simulink model "DC_observer_R2018a"  (R2018a)
settings: Solver=VariableStepAuto  StartTime=0.0  StopTime=2  MaxStep=1e-4  RelTol=1e-3
values from neighbouring files (symbols this model uses):
  A = [ -(k*gr)^2/(J*R)-b/J, 0 ... (first row only)    [DC_statespace.m]    (also in DC_statespace_facit.m; DC_statespace_observer.m)
  b = 20    [DC_statespace.m]    (also in DC_statespace_facit.m; DC_statespace_observer.m = B(1,1))
  B = [k*gr/(J*R) ... (first row only)    [DC_statespace.m]    (also in DC_statespace_facit.m; DC_statespace_observer.m)
  C = [0, 1]    [DC_statespace.m]    (also in DC_statespace_facit.m; DC_statespace_observer.m)
  gr = 200    [DC_statespace.m]    (also in DC_statespace_facit.m; DC_statespace_observer.m)
  J = 50*1.5^2    (= 112.5)    [DC_statespace.m]    (also in DC_statespace_facit.m; DC_statespace_observer.m)
  K = [k1;k2]    [DC_statespace_observer.m]
  k = Vmax / gr / (speed_max*pi/180)    (= 0.954929658551)    [DC_statespace.m]    (also in DC_statespace_facit.m; DC_statespace_observer.m)
  L = 4e-3    (= 0.004)    [DC_statespace.m]    (also in DC_statespace_facit.m; DC_statespace_observer.m)
  l_0 = 1.0/dcgain(cl_ss)    [DC_statespace.m]    (also in DC_statespace_facit.m; DC_statespace_observer.m)
  Lv = place(A, B, pd)    [DC_statespace.m]    (also in DC_statespace_facit.m; DC_statespace_observer.m = acker(A, B, pd))
  R = 5    [DC_statespace.m]    (also in DC_statespace_facit.m; DC_statespace_observer.m)
  Vmax = 400    [DC_statespace.m]    (also in DC_statespace_facit.m; DC_statespace_observer.m)
settings Model: Creator=kjartan  LastModifiedBy=kjartan
settings DataIOCC: ReturnWorkspaceOutputs=on
settings DebuggingCC: SFMachineParentedDataDiag=error
settings SFSimCC: SimUseLocalCustomCode=on
settings RTWCC: RTWUseLocalCustomCode=on

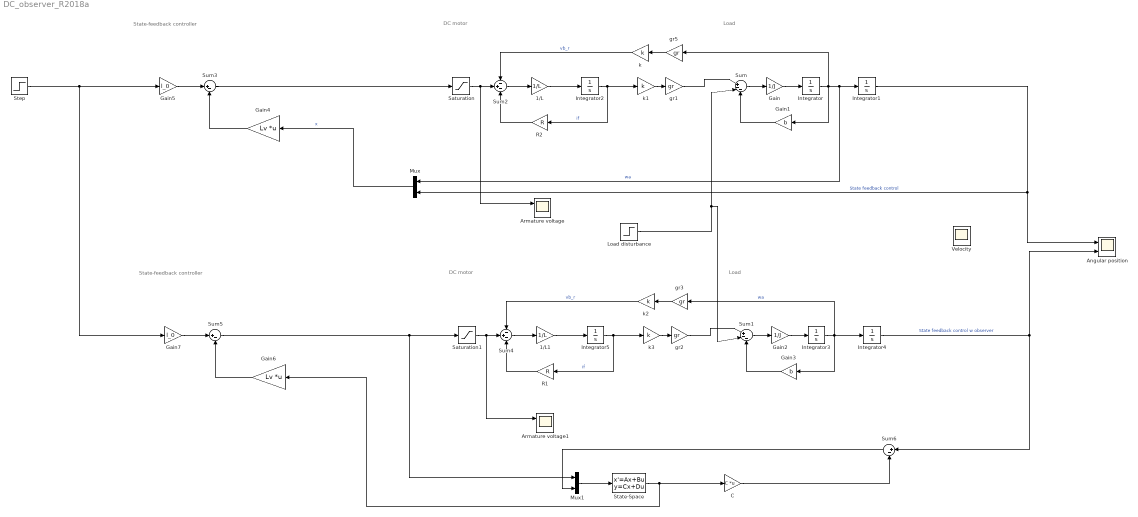
== system DC_observer_R2018a ==
  note: State-feedback controller
  note: Load
  note: DC motor
  note: Load
  note: DC motor
  note: State-feedback controller
  1/L : Gain  Gain=1/L
  1/L1 : Gain  Gain=1/L
  Angular position : Scope  NumInputPorts=2
  Armature voltage : Scope  NumInputPorts=2
  Armature voltage1 : Scope  NumInputPorts=2
  C : Gain  Gain=C  Multiplication=Matrix(K*u) (u vector)
  Gain : Gain  Gain=1/J
  Gain1 : Gain  Gain=b
  Gain2 : Gain  Gain=1/J
  Gain3 : Gain  Gain=b
  Gain4 : Gain  Gain=Lv  Multiplication=Matrix(K*u)
  Gain5 : Gain  Gain=l_0
  Gain6 : Gain  Gain=Lv  Multiplication=Matrix(K*u)
  Gain7 : Gain  Gain=l_0
  Integrator{,1..5} (6 alike) : Integrator
  Load disturbance : Step  After=1000  SampleTime=0
  Mux : Mux  Inputs=2
  Mux1 : Mux  Inputs=2
  R1 : Gain  Gain=R
  R2 : Gain  Gain=R
  Saturation : Saturate  UpperLimit=Vmax  LowerLimit=-Vmax
  Saturation1 : Saturate  UpperLimit=Vmax  LowerLimit=-Vmax
  State-Space : StateSpace  A=A  B=[B K]  C=eye(2)  D=zeros(2,2)  InitialCondition=0
  Step : Step  Time=0  After=0.1  SampleTime=0
  Sum : Sum  Inputs=|+--
  Sum1 : Sum  Inputs=|+--
  Sum2 : Sum  Inputs=-+-
  Sum3 : Sum  Inputs=|+-
  Sum4 : Sum  Inputs=-+-
  Sum5 : Sum  Inputs=|+-
  Sum6 : Sum  Inputs=|+-
  Velocity : Scope  NumInputPorts=2
  gr{1..3,5} (4 alike) : Gain  Gain=gr
  k{,1..3} (4 alike) : Gain  Gain=k
  wires:
  gr5/1 -> k/1
  R2/1 -> Sum2/3
  Integrator2/1 -> R2/1, k1/1  "if"
  Sum2/1 -> 1/L/1
  k1/1 -> gr1/1
  1/L/1 -> Integrator2/1
  k/1 -> Sum2/1  "vb_r"
  gr1/1 -> Sum/1
  Gain/1 -> Integrator/1
  Integrator/1 -> Gain1/1, gr5/1, Mux/1, Integrator1/1  "wa"
  Integrator1/1 -> Mux/2, Angular position/1  "State feedback control"
  Sum/1 -> Gain/1
  Gain1/1 -> Sum/3
  Load disturbance/1 -> Sum1/2, Sum/2
  Saturation/1 -> Armature voltage/1, Sum2/2
  Gain5/1 -> Sum3/1
  Mux/1 -> Gain4/1  "x"
  Gain4/1 -> Sum3/2
  Sum3/1 -> Saturation/1
  Integrator3/1 -> Gain3/1, gr3/1, Integrator4/1  "wa"
  gr3/1 -> k2/1
  Gain6/1 -> Sum5/2
  gr2/1 -> Sum1/1
  Integrator5/1 -> R1/1, k3/1  "if"
  Saturation1/1 -> Armature voltage1/1, Sum4/2
  Sum5/1 -> Mux1/1, Saturation1/1
  Sum4/1 -> 1/L1/1
  Integrator4/1 -> Angular position/2, Sum6/1  "State feedback control w observer"
  1/L1/1 -> Integrator5/1
  Gain2/1 -> Integrator3/1
  Gain3/1 -> Sum1/3
  k3/1 -> gr2/1
  k2/1 -> Sum4/1  "vb_r"
  R1/1 -> Sum4/3
  Sum1/1 -> Gain2/1
  Step/1 -> Gain7/1, Gain5/1
  Gain7/1 -> Sum5/1
  State-Space/1 -> Gain6/1, C/1
  C/1 -> Sum6/2
  Mux1/1 -> State-Space/1
  Sum6/1 -> Mux1/2
